simulink model "LaneFollowingDecisionLogic"  (R2022b)
settings: Solver=FixedStepDiscrete  StartTime=0.0  StopTime=10.0  RelTol=1e-3  SampleTimeConstraint=STIndependent  EnableMultiTasking=on
undefined symbols (not defined in the file): LaneWidth, posSelector
settings Model: Creator=The MathWorks, Inc.  LastModifiedBy=The MathWorks, Inc.
settings SolverCC: AlgebraicLoopSolver=TrustRegion
settings OptimizationCC: DefaultParameterBehavior=Inlined  InlineInvariantSignals=on  EnhancedBackFolding=on  PassReuseOutputArgsAs=Individual arguments  ZeroExternalMemoryAtStartup=off  ZeroInternalMemoryAtStartup=off  EfficientFloat2IntCast=on  OptimizeBlockOrder=speed  DifferentSizesBufferReuse=on  OptimizationCustomize=off  EfficientTunableParamExpr=on
settings DebuggingCC: ParameterTunabilityLossMsg=error  UnconnectedInputMsg=warning  UnconnectedOutputMsg=warning  UnconnectedLineMsg=warning  ModelReferenceSymbolNameMessage=none  SFMachineParentedDataDiag=warning
settings HardwareCC: ProdLongLongMode=on
settings ModelReferenceCC: EnableRefExpFcnMdlSchedulingChecks=on  PropagateVarSize=During execution
settings RTWCC: Description=Embedded Coder  SystemTargetFile=ert.tlc  TemplateMakefile=ert_default_tmf  RTWVerbose=off  BuildConfiguration=Faster Runs  CodeExecutionProfiling=on  CodeProfilingSaveOptions=AllData  TargetLang=C++  DLArmComputeVersion=19.05
settings CodeAppCC: ForceParamTrailComments=on  IgnoreCustomStorageClasses=off  OperatorAnnotations=on  SimulinkDataObjDesc=on  SFDataObjDesc=on  CustomSymbolStrGlobalVar=$N$M  CustomSymbolStrType=$N$M_T  CustomSymbolStrFcn=APV_$N$M$F  CustomSymbolStrMacro=$N$M  InsertBlockDesc=on
settings ERTTargetCC: TargetLangStandard=C++03 (ISO)  GenerateSampleERTMain=on  CombineSignalStateStructs=on  CodeInterfacePackaging=C++ class  SupportVariableSizeSignals=on  CastingMode=Standards  InlinedParameterPlacement=NonHierarchical  RootIOFormat=Structure reference  ERTCustomFileTemplate=example_file_process.tlc

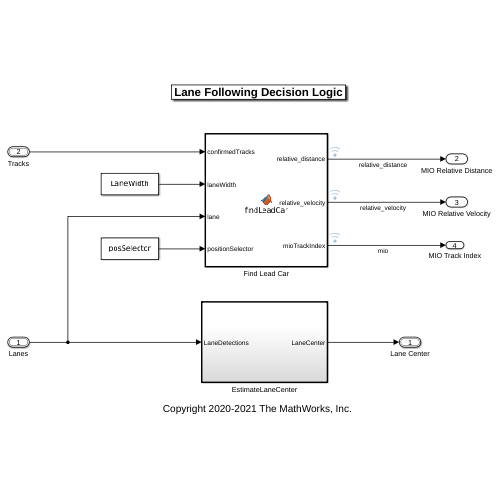
[thumbnail: Simulink's stored preview of the top-level diagram]
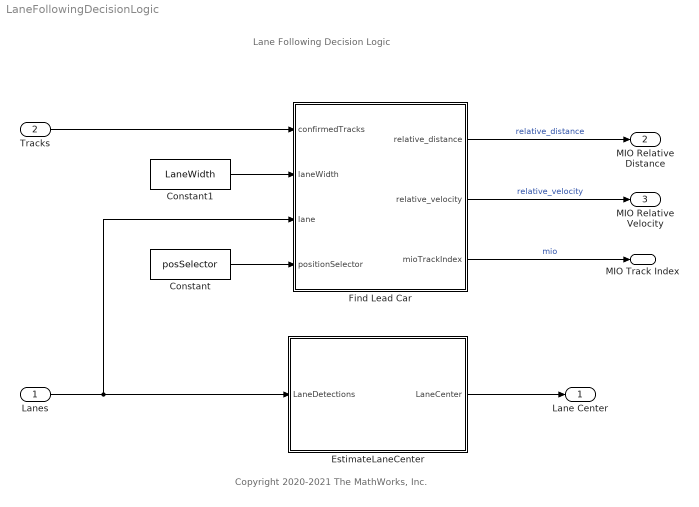
== system LaneFollowingDecisionLogic ==
  note: Lane Following Decision Logic
  note: Copyright 2020-2021 The MathWorks, Inc.
  Lanes : Inport  OutDataTypeStr=Bus: LaneSensor  PortDimensions=[1 1]
  Tracks : Inport  Port=2  OutDataTypeStr=Bus: BusTrackerJPDA  PortDimensions=[1 1]  BusOutputAsStruct=on
  Constant : Constant  Value=posSelector
  Constant1 : Constant  Value=LaneWidth
  EstimateLaneCenter : Subsystem  TreatAsAtomicUnit=on  VariantControl=v2
      settings: RTWFileNameOpts=Use function name
  Find Lead Car : MATLAB Function  TreatAsAtomicUnit=on
  Lane Center : Outport  OutDataTypeStr=Bus: BusLaneCenter
  MIO Relative Distance : Outport  Port=2
  MIO Relative Velocity : Outport  Port=3
  MIO Track Index : Outport  Port=4  PortDimensions=1  VectorParamsAs1DForOutWhenUnconnected=off  BusOutputAsStruct=on
  wires:
  Find Lead Car/3(mioTrackIndex) -> MIO Track Index/1  "mio"
  Find Lead Car/2(relative_velocity) -> MIO Relative Velocity/1  "relative_velocity"
  Constant/1 -> Find Lead Car/4(positionSelector)
  Tracks/1 -> Find Lead Car/1(confirmedTracks)
  Find Lead Car/1(relative_distance) -> MIO Relative Distance/1  "relative_distance"
  Constant1/1 -> Find Lead Car/2(laneWidth)
  EstimateLaneCenter/1(LaneCenter) -> Lane Center/1
  Lanes/1 -> Find Lead Car/3(lane), EstimateLaneCenter/1(LaneDetections)

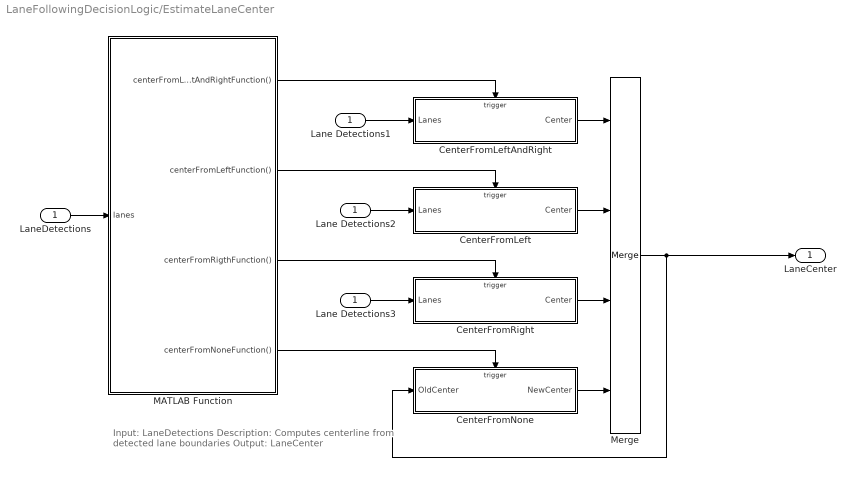
== system LaneFollowingDecisionLogic/EstimateLaneCenter ==
  note: Input: LaneDetections
      | Description: Computes centerline from detected lane boundaries
      | Output: LaneCenter
  LaneDetections : Inport
  CenterFromLeft : Subsystem  TreatAsAtomicUnit=on
  CenterFromLeftAndRight : Subsystem  TreatAsAtomicUnit=on
  CenterFromNone : Subsystem  TreatAsAtomicUnit=on
  CenterFromRight : Subsystem  TreatAsAtomicUnit=on
  Lane Detections1 : InportShadow
  Lane Detections2 : InportShadow
  Lane Detections3 : InportShadow
  MATLAB Function : MATLAB Function  TreatAsAtomicUnit=on
  Merge : Merge  Inputs=4
  LaneCenter : Outport
  wires:
  CenterFromRight/1(Center) -> Merge/3
  Lane Detections2/1 -> CenterFromLeft/1(Lanes)
  Lane Detections3/1 -> CenterFromRight/1(Lanes)
  MATLAB Function/2(centerFromLeftFunction()) -> CenterFromLeft/Trigger
  CenterFromNone/1(NewCenter) -> Merge/4
  MATLAB Function/1(centerFromLeftAndRightFunction()) -> CenterFromLeftAndRight/Trigger
  Merge/1 -> CenterFromNone/1(OldCenter), LaneCenter/1
  CenterFromLeftAndRight/1(Center) -> Merge/1
  LaneDetections/1 -> MATLAB Function/1(lanes)
  Lane Detections1/1 -> CenterFromLeftAndRight/1(Lanes)
  MATLAB Function/3(centerFromRigthFunction()) -> CenterFromRight/Trigger
  MATLAB Function/4(centerFromNoneFunction()) -> CenterFromNone/Trigger
  CenterFromLeft/1(Center) -> Merge/2

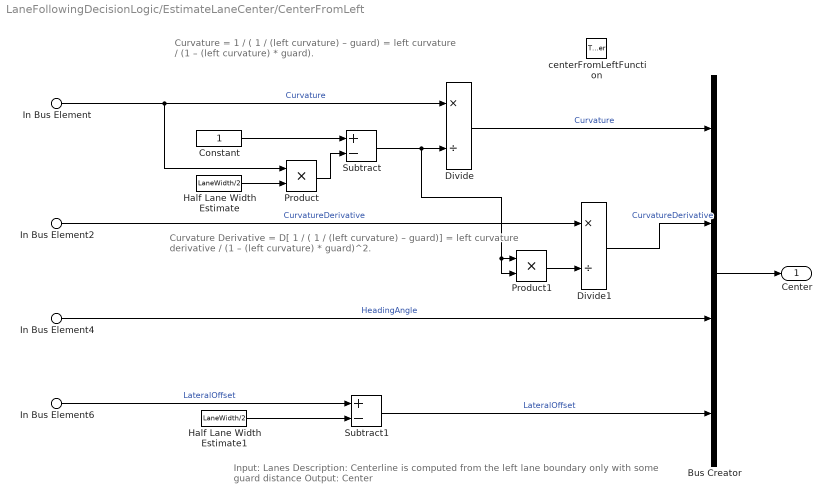
== system LaneFollowingDecisionLogic/EstimateLaneCenter/CenterFromLeft ==
  note: Curvature Derivative
      | = D[ 1 / ( 1 / (left curvature) – guard)]
      | = left curvature derivative / (1 – (left curvature) * guard)^2.
  note: Curvature
      | = 1 / ( 1 / (left curvature) – guard)
      | = left curvature / (1 – (left curvature) * guard).
  note: Input: Lanes
      | Description: Centerline is computed from the left lane boundary only with some guard distance
      | Output: Center
  In Bus Element : Inport  PortName=Lanes  Element=Left.Curvature
  In Bus Element2 : Inport  PortName=Lanes  Element=Left.CurvatureDerivative
  In Bus Element4 : Inport  PortName=Lanes  Element=Left.HeadingAngle
  In Bus Element6 : Inport  PortName=Lanes  Element=Left.LateralOffset
  centerFromLeftFunction : TriggerPort  TriggerType=function-call  VariantControl=Variant
  Bus Creator : BusCreator  Inputs=4
  Constant : Constant  OutDataTypeStr=Inherit: Inherit via back propagation
  Divide : Product  Inputs=*/
  Divide1 : Product  Inputs=*/
  Half Lane Width Estimate : Constant  Value=LaneWidth/2  OutDataTypeStr=Inherit: Inherit via back propagation
  Half Lane Width Estimate1 : Constant  Value=LaneWidth/2  OutDataTypeStr=Inherit: Inherit via back propagation
  Product : Product
  Product1 : Product
  Subtract : Sum  Inputs=+-
  Subtract1 : Sum  Inputs=+-
  Center : Outport  VectorParamsAs1DForOutWhenUnconnected=off
  wires:
  Product/1 -> Subtract/2
  Half Lane Width Estimate1/1 -> Subtract1/2
  In Bus Element6/1 -> Subtract1/1  "LateralOffset"
  Product1/1 -> Divide1/2
  In Bus Element2/1 -> Divide1/1  "CurvatureDerivative"
  Constant/1 -> Subtract/1
  Half Lane Width Estimate/1 -> Product/2
  Subtract/1 -> Divide/2, Product1/1, Product1/2
  In Bus Element/1 -> Divide/1, Product/1  "Curvature"
  Subtract1/1 -> Bus Creator/4  "LateralOffset"
  In Bus Element4/1 -> Bus Creator/3  "HeadingAngle"
  Divide/1 -> Bus Creator/1  "Curvature"
  Divide1/1 -> Bus Creator/2  "CurvatureDerivative"
  Bus Creator/1 -> Center/1

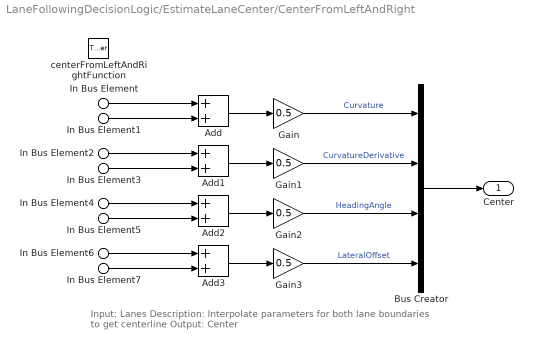
== system LaneFollowingDecisionLogic/EstimateLaneCenter/CenterFromLeftAndRight ==
  note: Input: Lanes
      | Description: Interpolate parameters for both lane boundaries to get centerline
      | Output: Center
  In Bus Element : Inport  PortName=Lanes  Element=Left.Curvature
  In Bus Element2 : Inport  PortName=Lanes  Element=Left.CurvatureDerivative
  In Bus Element4 : Inport  PortName=Lanes  Element=Left.HeadingAngle
  In Bus Element6 : Inport  PortName=Lanes  Element=Left.LateralOffset
  In Bus Element1 : Inport  PortName=Lanes  Element=Right.Curvature
  In Bus Element3 : Inport  PortName=Lanes  Element=Right.CurvatureDerivative
  In Bus Element5 : Inport  PortName=Lanes  Element=Right.HeadingAngle
  In Bus Element7 : Inport  PortName=Lanes  Element=Right.LateralOffset
  centerFromLeftAndRightFunction : TriggerPort  TriggerType=function-call  VariantControl=Variant
  Add{,1..3} (4 alike) : Sum
  Bus Creator : BusCreator  Inputs=4
  Gain{,1..3} (4 alike) : Gain  Gain=0.5
  Center : Outport  VectorParamsAs1DForOutWhenUnconnected=off
  wires:
  In Bus Element6/1 -> Add3/1
  In Bus Element7/1 -> Add3/2
  In Bus Element5/1 -> Add2/2
  In Bus Element4/1 -> Add2/1
  In Bus Element3/1 -> Add1/2
  In Bus Element2/1 -> Add1/1
  In Bus Element1/1 -> Add/2
  In Bus Element/1 -> Add/1
  Bus Creator/1 -> Center/1
  Gain3/1 -> Bus Creator/4  "LateralOffset"
  Add3/1 -> Gain3/1
  Gain2/1 -> Bus Creator/3  "HeadingAngle"
  Add2/1 -> Gain2/1
  Gain1/1 -> Bus Creator/2  "CurvatureDerivative"
  Add1/1 -> Gain1/1
  Gain/1 -> Bus Creator/1  "Curvature"
  Add/1 -> Gain/1

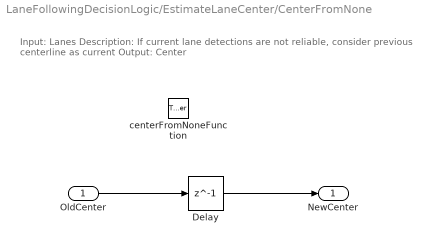
== system LaneFollowingDecisionLogic/EstimateLaneCenter/CenterFromNone ==
  note: Input: Lanes
      | Description: If current lane detections are not reliable, consider previous centerline as current
      | Output: Center
  OldCenter : Inport
      settings: LatchInputForFeedbackSignals=on
  centerFromNoneFunction : TriggerPort  TriggerType=function-call  VariantControl=Variant
  Delay : Delay  DelayLength=1
  NewCenter : Outport  VectorParamsAs1DForOutWhenUnconnected=off
  wires:
  OldCenter/1 -> Delay/1
  Delay/1 -> NewCenter/1

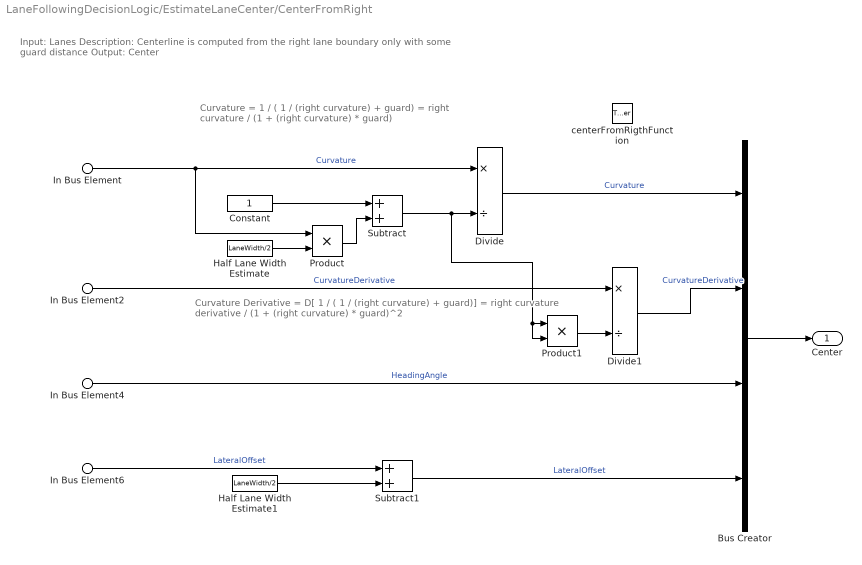
== system LaneFollowingDecisionLogic/EstimateLaneCenter/CenterFromRight ==
  note: Curvature Derivative
      | = D[ 1 / ( 1 / (right curvature) + guard)]
      | = right curvature derivative / (1 + (right curvature) * guard)^2
  note: Curvature
      | = 1 / ( 1 / (right curvature) + guard)
      | = right curvature / (1 + (right curvature) * guard)
  note: Input: Lanes
      | Description: Centerline is computed from the right lane boundary only with some guard distance
      | Output: Center
  In Bus Element : Inport  PortName=Lanes  Element=Right.Curvature
  In Bus Element2 : Inport  PortName=Lanes  Element=Right.CurvatureDerivative
  In Bus Element4 : Inport  PortName=Lanes  Element=Right.HeadingAngle
  In Bus Element6 : Inport  PortName=Lanes  Element=Right.LateralOffset
  centerFromRigthFunction : TriggerPort  TriggerType=function-call  VariantControl=Variant
  Bus Creator : BusCreator  Inputs=4
  Constant : Constant  OutDataTypeStr=Inherit: Inherit via back propagation
  Divide : Product  Inputs=*/
  Divide1 : Product  Inputs=*/
  Half Lane Width Estimate : Constant  Value=LaneWidth/2  OutDataTypeStr=Inherit: Inherit via back propagation
  Half Lane Width Estimate1 : Constant  Value=LaneWidth/2  OutDataTypeStr=Inherit: Inherit via back propagation
  Product : Product
  Product1 : Product
  Subtract : Sum
  Subtract1 : Sum
  Center : Outport  VectorParamsAs1DForOutWhenUnconnected=off
  wires:
  Half Lane Width Estimate/1 -> Product/2
  Product/1 -> Subtract/2
  Constant/1 -> Subtract/1
  Subtract/1 -> Divide/2, Product1/1, Product1/2
  In Bus Element/1 -> Divide/1, Product/1  "Curvature"
  Bus Creator/1 -> Center/1
  Subtract1/1 -> Bus Creator/4  "LateralOffset"
  Divide/1 -> Bus Creator/1  "Curvature"
  In Bus Element6/1 -> Subtract1/1  "LateralOffset"
  Half Lane Width Estimate1/1 -> Subtract1/2
  In Bus Element4/1 -> Bus Creator/3  "HeadingAngle"
  Product1/1 -> Divide1/2
  Divide1/1 -> Bus Creator/2  "CurvatureDerivative"
  In Bus Element2/1 -> Divide1/1  "CurvatureDerivative"

== matlab function LaneFollowingDecisionLogic/Find Lead Car ==
  data: confirmedTracks input; laneWidth input; relative_distance output size=[1 1]; relative_velocity output size=[1 1]; lane input; mioTrackIndex output; positionSelector input
function [relative_distance,relative_velocity,mioTrackIndex] = findLeadCar(confirmedTracks, laneWidth, lane, positionSelector)
% This function finds the lead car: a car in front of the ego car that
% satisfies all the criteria below:
% * Within the ego car's lane.
% * In front of the ego car.
% * Closest to the ego car.

% Note: If you change state definition, change the following:
%       State = [x;vx;y;vy;z;vz] (3D constant velocity)
numStates = 6;
numTracks = confirmedTracks.NumTracks;
% Initialize outputs and parameters
egoVehicleIdx = uint8(1);
maxX = cast(1000, 'like', confirmedTracks.Tracks(egoVehicleIdx).State);  % Far enough forward so that no track is expected to exceed this distance
mioTrackIndex = 0;

% If lane detection is not available, the ego car is assumed to be located
% in the middle of its lane. The lane width is assumed to be 3.6m, typical
% highway lane width.
    
halfLaneWidth = laneWidth/2;

if lane.Left.Strength > 0.01
    lb = [lane.Left.CurvatureDerivative/6,...
        lane.Left.Curvature/2,...
        lane.Left.HeadingAngle,...
        lane.Left.LateralOffset];
else
    lb = single([0,0,0,halfLaneWidth]);
end

if lane.Right.Strength > 0.01
    rb = [lane.Right.CurvatureDerivative/6,...
        lane.Right.Curvature/2,...
        lane.Right.HeadingAngle,...
        lane.Right.LateralOffset];
else
    rb = single([0,0,0,-halfLaneWidth]);    
end


for i = 1:numTracks
    position = positionSelector * confirmedTracks.Tracks(i).State;
    relative_distance = position(uint8(1)); % Longitudinal position of the track relative to ego
    y = single(position(uint8(2))); % Lateral position of the track relative to ego
    
    % Checking for MIO if the track is in free space
    if relative_distance < maxX && relative_distance > 2 

        yleftLane  = polyval(lb,relative_distance); % lateral position of left lane
        yrightLane = polyval(rb,relative_distance); % lateral position of right lane
        
        % Find a new lead car
        if (yrightLane <= y) && (y <= yleftLane)
            maxX = relative_distance;
            mioTrackIndex = i;
        end
    end
end

if mioTrackIndex>0
    mioState = confirmedTracks.Tracks(mioTrackIndex).State;
else
    mioState = 10000*ones(numStates,1,'like',confirmedTracks.Tracks(egoVehicleIdx).State);
end

% Output:
relative_distance = mioState(uint8(1));    % Longitudinal position of the lead car
relative_velocity = mioState(uint8(2));   % Longitudinal velocity of the lead car

== matlab function LaneFollowingDecisionLogic/EstimateLaneCenter/MATLAB Function ==
  data: lanes input
  events: centerFromLeftAndRightFunction output FUNCTION_CALL_EVENT; centerFromLeftFunction output FUNCTION_CALL_EVENT; centerFromRigthFunction output FUNCTION_CALL_EVENT; centerFromNoneFunction output FUNCTION_CALL_EVENT
function fcn(lanes)

leftStrength  = lanes.Left.Strength;
rightStrength = lanes.Right.Strength;

if (leftStrength > 0) && (rightStrength > 0)
   centerFromLeftAndRightFunction();
   
elseif leftStrength > 0
    centerFromLeftFunction();
    
elseif rightStrength > 0
    centerFromRigthFunction();
    
else
    centerFromNoneFunction();
end
